simulink model "Flight_Control"  (Simulink 9.0)
settings: Solver=FixedStepDiscrete  StartTime=0.0  StopTime=tsim  FixedStep=te  RelTol=1e-3
values from neighbouring files (symbols this model uses):
  Kb_Pitch = 4    [Flight_Control_parameters.m]
  Kb_Roll = 4    [Flight_Control_parameters.m]
  Kb_Yaw = 4    [Flight_Control_parameters.m]
  Kd_Pitch = 0.037    [Flight_Control_parameters.m]
  Kd_Roll = 0.037    [Flight_Control_parameters.m]
  Kd_Yaw = 0.1    [Flight_Control_parameters.m]
  Ki_Pitch = 5    [Flight_Control_parameters.m]
  Ki_Roll = 5    [Flight_Control_parameters.m]
  Ki_Yaw = 5    [Flight_Control_parameters.m]
  Kp_Pitch = 3.84    [Flight_Control_parameters.m]
  Kp_pitch_angle = 4    [Flight_Control_parameters.m]
  Kp_Roll = 3.84    [Flight_Control_parameters.m]
  Kp_roll_angle = 4    [Flight_Control_parameters.m]
  Kp_Yaw = 8.16    [Flight_Control_parameters.m]
  te = 0.01    [Flight_Control_parameters.m]
undefined symbols (not defined in the file or in its folder): DiscIntNeverNeededParam
libraries: simulink x3
settings Model: Creator=sam  LastModifiedBy=William  ExtModeTrigDuration=2
settings DataIOCC: SaveFormat=Dataset
settings OptimizationCC: DefaultParameterBehavior=Inlined  DefaultUnderspecifiedDataType=single  PassReuseOutputArgsThreshold=0  LifeSpan=auto  MaxStackSize=64
settings DebuggingCC: UnderspecifiedInitializationDetection=Simplified  MergeDetectMultiDrivingBlocksExec=error  ParameterPrecisionLossMsg=none  ParameterTunabilityLossMsg=error
settings HardwareCC: ProdBitPerPointer=64  ProdBitPerSizeT=64  ProdBitPerPtrDiffT=64  ProdLargestAtomicFloat=Float  ProdIntDivRoundTo=Zero  ProdEndianess=LittleEndian  ProdWordSize=64  ProdHWDeviceType=Intel->x86-64 (Windows64)
settings ModelReferenceCC: PropagateSignalLabelsOutOfModel=on
settings SFSimCC: MATLABDynamicMemAlloc=off
settings RTWCC: GenerateReport=on  Toolchain=Arduino ARM  BuildConfiguration=Faster Runs  LaunchReport=on  RTWCompilerOptimization=on
settings CodeAppCC: ForceParamTrailComments=on  MaxIdLength=95  OperatorAnnotations=on  MATLABSourceComments=on
settings ConfigComp: CovScope=Subsystem  CovPath=Flight_Control  CovSaveName=covdata_decision  CovMetricSettings=dcmw  CovHTMLOptions=-sRT=1 -sVT=0 -aTS=1 -bRG=1 -bTC=1 -hTR=0 -nFC=0 -nFD=1 -scm=1 -bcm=1 -xEv=0 -xEM=0  CovNameIncrementing=on  CovOutputDir=../reports/slcov_output/$ModelName$

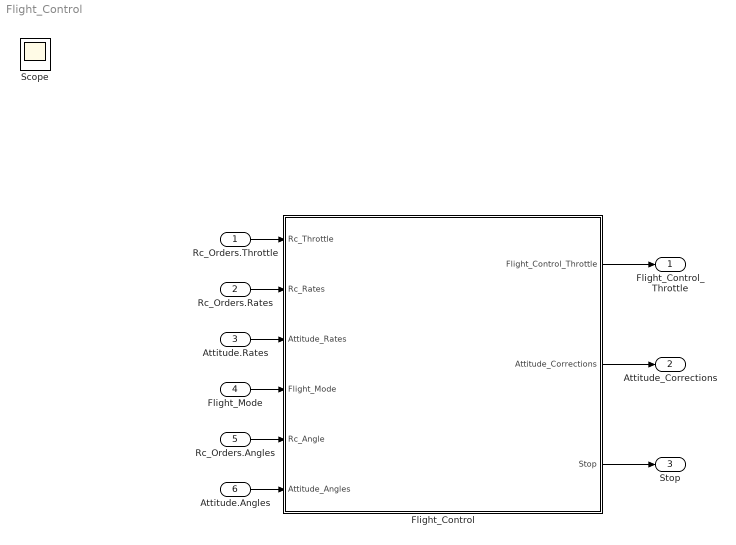
== system Flight_Control ==
  Rc_Orders.Throttle : Inport  OutDataTypeStr=single  PortDimensions=1
  Rc_Orders.Rates : Inport  Port=2  OutDataTypeStr=single  PortDimensions=3
  Attitude.Rates : Inport  Port=3  OutDataTypeStr=single  PortDimensions=3
  Flight_Mode : Inport  Port=4  OutDataTypeStr=uint8
  Rc_Orders.Angles : Inport  Port=5  OutDataTypeStr=single  PortDimensions=2
  Attitude.Angles : Inport  Port=6  OutDataTypeStr=single  PortDimensions=2
  Flight_Control : Subsystem
  Flight_Control_Throttle : Outport  OutDataTypeStr=single  PortDimensions=1
  Attitude_Corrections : Outport  Port=2  OutDataTypeStr=single  PortDimensions=3
  Stop : Outport  Port=3  OutDataTypeStr=boolean  PortDimensions=1
  Scope : Scope
  wires:
  Flight_Control/1(Flight_Control_Throttle) -> Flight_Control_Throttle/1
  Flight_Control/2(Attitude_Corrections) -> Attitude_Corrections/1
  Flight_Control/3(Stop) -> Stop/1
  Rc_Orders.Throttle/1 -> Flight_Control/1(Rc_Throttle)
  Rc_Orders.Rates/1 -> Flight_Control/2(Rc_Rates)
  Attitude.Rates/1 -> Flight_Control/3(Attitude_Rates)
  Flight_Mode/1 -> Flight_Control/4(Flight_Mode)
  Rc_Orders.Angles/1 -> Flight_Control/5(Rc_Angle)
  Attitude.Angles/1 -> Flight_Control/6(Attitude_Angles)

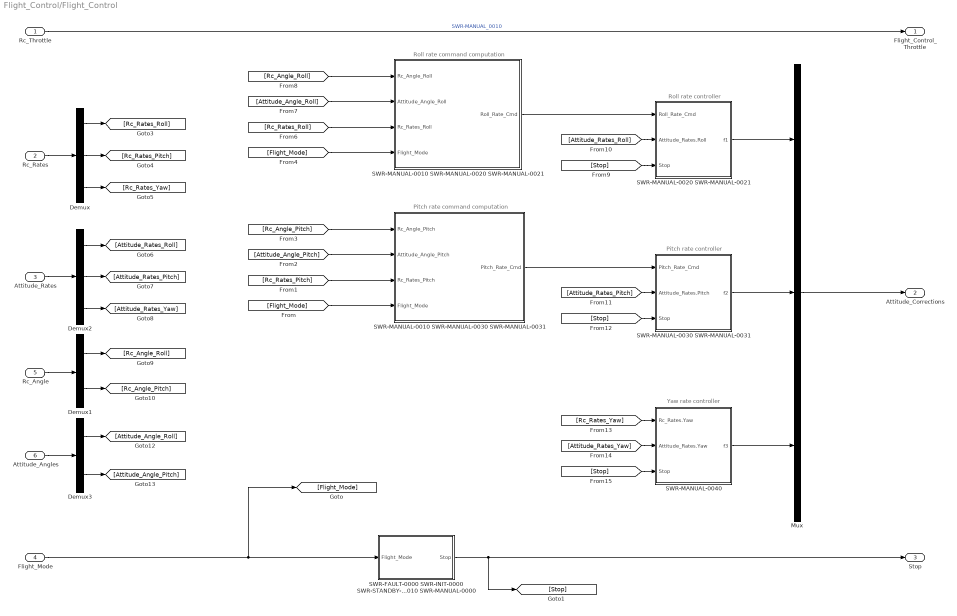
== system Flight_Control/Flight_Control ==
  note: Roll rate controller
  note: Pitch rate controller
  note: Yaw rate controller
  note: Roll rate command computation
  note: Pitch rate command computation
  Rc_Throttle : Inport  PortDimensions=1
  Rc_Rates : Inport  Port=2  PortDimensions=3
  Attitude_Rates : Inport  Port=3  PortDimensions=3
  Flight_Mode : Inport  Port=4  PortDimensions=1
  Rc_Angle : Inport  Port=5  PortDimensions=2
  Attitude_Angles : Inport  Port=6  PortDimensions=2
  Demux : Demux  Outputs=3
  Demux1 : Demux  Outputs=2
  Demux2 : Demux  Outputs=3
  Demux3 : Demux  Outputs=2
  Mux : Mux  Inputs=3
  SWR-FAULT-0000 SWR-INIT-0000 SWR-STANDBY-0000 SWR-STANDBY-0010 SWR-MANUAL-0000 : Subsystem
  "SWR-MANUAL-0010 SWR-MANUAL-0020 SWR-MANUAL-0021 " : Subsystem
  "SWR-MANUAL-0010 SWR-MANUAL-0030 SWR-MANUAL-0031 " : Subsystem
  SWR-MANUAL-0020 SWR-MANUAL-0021 : Subsystem
  SWR-MANUAL-0030 SWR-MANUAL-0031 : Subsystem
  SWR-MANUAL-0040 : Subsystem
  Flight_Control_Throttle : Outport  PortDimensions=1
  Attitude_Corrections : Outport  Port=2  PortDimensions=3
  Stop : Outport  Port=3  PortDimensions=1
  wires:
  Rc_Rates/1 -> Demux/1
  Attitude_Rates/1 -> Demux2/1
  Demux/1 -> [Rc_Rates_Roll]
  Demux/2 -> [Rc_Rates_Pitch]
  Demux/3 -> [Rc_Rates_Yaw]
  Demux2/3 -> [Attitude_Rates_Yaw]
  Demux2/1 -> [Attitude_Rates_Roll]
  Demux2/2 -> [Attitude_Rates_Pitch]
  [Attitude_Rates_Pitch] -> SWR-MANUAL-0030 SWR-MANUAL-0031/2(Attitude_Rates.Pitch)
  Mux/1 -> Attitude_Corrections/1
  SWR-FAULT-0000 SWR-INIT-0000 SWR-STANDBY-0000 SWR-STANDBY-0010 SWR-MANUAL-0000/1("Stop ") -> [Stop], Stop/1
  Rc_Throttle/1 -> Flight_Control_Throttle/1  "SWR-MANUAL_0010"
  [Stop] -> SWR-MANUAL-0020 SWR-MANUAL-0021/3(Stop)
  [Stop] -> SWR-MANUAL-0030 SWR-MANUAL-0031/3(Stop)
  SWR-MANUAL-0040/1(f3) -> Mux/3
  Rc_Angle/1 -> Demux1/1
  Demux1/1 -> [Rc_Angle_Roll]
  Demux1/2 -> [Rc_Angle_Pitch]
  Attitude_Angles/1 -> Demux3/1
  Demux3/2 -> [Attitude_Angle_Pitch]
  Demux3/1 -> [Attitude_Angle_Roll]
  [Attitude_Rates_Roll] -> SWR-MANUAL-0020 SWR-MANUAL-0021/2(Attitude_Rates.Roll)
  Flight_Mode/1 -> SWR-FAULT-0000 SWR-INIT-0000 SWR-STANDBY-0000 SWR-STANDBY-0010 SWR-MANUAL-0000/1(Flight_Mode), [Flight_Mode]
  SWR-MANUAL-0020 SWR-MANUAL-0021/1(f1) -> Mux/1
  SWR-MANUAL-0030 SWR-MANUAL-0031/1(f2) -> Mux/2
  [Rc_Rates_Yaw] -> SWR-MANUAL-0040/1(Rc_Rates.Yaw)
  [Attitude_Rates_Yaw] -> SWR-MANUAL-0040/2(Attitude_Rates.Yaw)
  [Stop] -> SWR-MANUAL-0040/3(Stop)
  "SWR-MANUAL-0010 SWR-MANUAL-0020 SWR-MANUAL-0021 "/1(Roll_Rate_Cmd) -> SWR-MANUAL-0020 SWR-MANUAL-0021/1(Roll_Rate_Cmd)
  [Rc_Angle_Roll] -> "SWR-MANUAL-0010 SWR-MANUAL-0020 SWR-MANUAL-0021 "/1(Rc_Angle_Roll)
  [Attitude_Angle_Roll] -> "SWR-MANUAL-0010 SWR-MANUAL-0020 SWR-MANUAL-0021 "/2(Attitude_Angle_Roll)
  [Flight_Mode] -> "SWR-MANUAL-0010 SWR-MANUAL-0020 SWR-MANUAL-0021 "/4(Flight_Mode)
  [Rc_Rates_Roll] -> "SWR-MANUAL-0010 SWR-MANUAL-0020 SWR-MANUAL-0021 "/3(Rc_Rates_Roll)
  "SWR-MANUAL-0010 SWR-MANUAL-0030 SWR-MANUAL-0031 "/1(Pitch_Rate_Cmd) -> SWR-MANUAL-0030 SWR-MANUAL-0031/1(Pitch_Rate_Cmd)
  [Rc_Angle_Pitch] -> "SWR-MANUAL-0010 SWR-MANUAL-0030 SWR-MANUAL-0031 "/1(Rc_Angle_Pitch)
  [Attitude_Angle_Pitch] -> "SWR-MANUAL-0010 SWR-MANUAL-0030 SWR-MANUAL-0031 "/2(Attitude_Angle_Pitch)
  [Rc_Rates_Pitch] -> "SWR-MANUAL-0010 SWR-MANUAL-0030 SWR-MANUAL-0031 "/3(Rc_Rates_Pitch)
  [Flight_Mode] -> "SWR-MANUAL-0010 SWR-MANUAL-0030 SWR-MANUAL-0031 "/4(Flight_Mode)

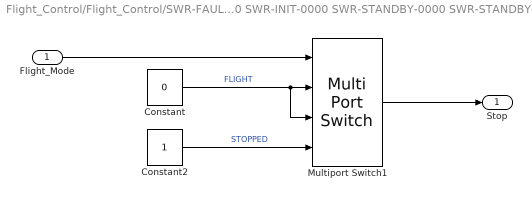
== system Flight_Control/Flight_Control/SWR-FAULT-0000 SWR-INIT-0000 SWR-STANDBY-0000 SWR-STANDBY-0010 SWR-MANUAL-0000 ==
  Flight_Mode : Inport  PortDimensions=1
  Constant : Constant  Value=0  OutDataTypeStr=boolean
  Constant2 : Constant  OutDataTypeStr=boolean
  Multiport Switch1 : MultiPortSwitch  DiagnosticForDefault=None
  "Stop " : Outport  PortDimensions=1
  wires:
  Constant/1 -> Multiport Switch1/3, Multiport Switch1/2  "FLIGHT"
  Flight_Mode/1 -> Multiport Switch1/1
  Multiport Switch1/1 -> "Stop "/1
  Constant2/1 -> Multiport Switch1/4  "STOPPED"

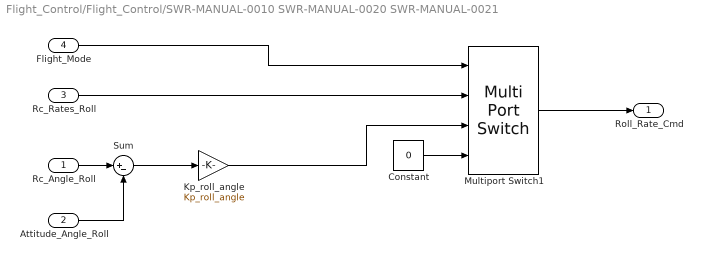
== system Flight_Control/Flight_Control/SWR-MANUAL-0010 SWR-MANUAL-0020 SWR-MANUAL-0021  ==
  Rc_Angle_Roll : Inport
  Attitude_Angle_Roll : Inport  Port=2
  Rc_Rates_Roll : Inport  Port=3
  Flight_Mode : Inport  Port=4
  Constant : Constant  Value=0  OutDataTypeStr=single
  Kp_roll_angle : Gain  Gain=Kp_roll_angle
  Multiport Switch1 : MultiPortSwitch  DiagnosticForDefault=None
  Sum : Sum  Inputs=|+-
  Roll_Rate_Cmd : Outport
  wires:
  Multiport Switch1/1 -> Roll_Rate_Cmd/1
  Kp_roll_angle/1 -> Multiport Switch1/3
  Rc_Angle_Roll/1 -> Sum/1
  Attitude_Angle_Roll/1 -> Sum/2
  Sum/1 -> Kp_roll_angle/1
  Flight_Mode/1 -> Multiport Switch1/1
  Rc_Rates_Roll/1 -> Multiport Switch1/2
  Constant/1 -> Multiport Switch1/4

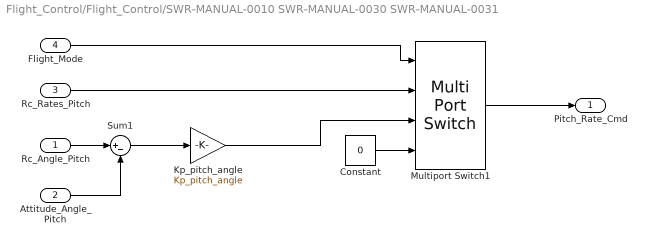
== system Flight_Control/Flight_Control/SWR-MANUAL-0010 SWR-MANUAL-0030 SWR-MANUAL-0031  ==
  Rc_Angle_Pitch : Inport
  Attitude_Angle_Pitch : Inport  Port=2
  Rc_Rates_Pitch : Inport  Port=3
  Flight_Mode : Inport  Port=4
  Constant : Constant  Value=0  OutDataTypeStr=single
  Kp_pitch_angle : Gain  Gain=Kp_pitch_angle
  Multiport Switch1 : MultiPortSwitch  DiagnosticForDefault=None
  Sum1 : Sum  Inputs=|+-
  Pitch_Rate_Cmd : Outport
  wires:
  Sum1/1 -> Kp_pitch_angle/1
  Rc_Angle_Pitch/1 -> Sum1/1
  Attitude_Angle_Pitch/1 -> Sum1/2
  Multiport Switch1/1 -> Pitch_Rate_Cmd/1
  Flight_Mode/1 -> Multiport Switch1/1
  Rc_Rates_Pitch/1 -> Multiport Switch1/2
  Kp_pitch_angle/1 -> Multiport Switch1/3
  Constant/1 -> Multiport Switch1/4

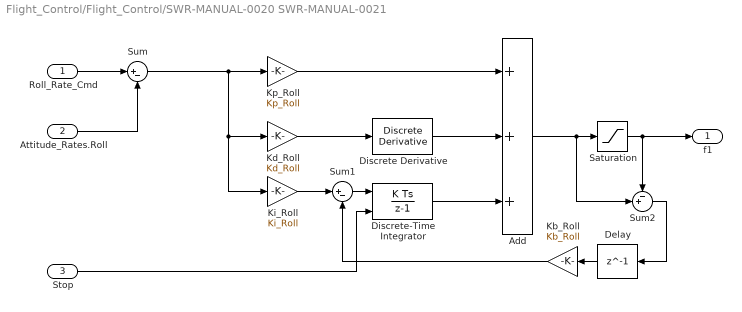
== system Flight_Control/Flight_Control/SWR-MANUAL-0020 SWR-MANUAL-0021 ==
  Roll_Rate_Cmd : Inport  PortDimensions=1
  Attitude_Rates.Roll : Inport  Port=2  PortDimensions=1
  Stop : Inport  Port=3  PortDimensions=1
  Add : Sum  Inputs=+++
  Delay : Delay  DelayLength=1  InitialCondition=0  SampleTime=te
  Discrete Derivative : simulink/Discrete/Discrete Derivative  gainval=1.0  ICPrevScaledInput=0.0  OutMin=[]  OutMax=[]  OutDataType=fixdt(1, 16)  OutScaling=2^-10  DoSatur=off
  Discrete-Time Integrator : DiscreteIntegrator  ExternalReset=level  InitialConditionSetting=State (most efficient)  SampleTime=te  UpperSaturationLimit=100  LowerSaturationLimit=-100  ICPrevOutput=DiscIntNeverNeededParam  ICPrevScaledInput=DiscIntNeverNeededParam
  Kb_Roll : Gain  Gain=Kb_Roll  ParamDataTypeStr=Inherit: Same as input
  Kd_Roll : Gain  Gain=Kd_Roll  ParamDataTypeStr=Inherit: Same as input
  Ki_Roll : Gain  Gain=Ki_Roll  ParamDataTypeStr=Inherit: Same as input
  Kp_Roll : Gain  Gain=Kp_Roll  ParamDataTypeStr=Inherit: Same as input
  Saturation : Saturate  UpperLimit=30  LowerLimit=-30
  Sum : Sum  Inputs=|+-
  Sum1 : Sum  Inputs=|+-
  Sum2 : Sum  Inputs=-+|
  f1 : Outport  PortDimensions=1
  wires:
  Add/1 -> Saturation/1, Sum2/2
  Roll_Rate_Cmd/1 -> Sum/1
  Attitude_Rates.Roll/1 -> Sum/2
  Sum/1 -> Kd_Roll/1, Ki_Roll/1, Kp_Roll/1
  Kp_Roll/1 -> Add/1
  Stop/1 -> Discrete-Time Integrator/2
  Discrete-Time Integrator/1 -> Add/3
  Discrete Derivative/1 -> Add/2
  Kd_Roll/1 -> Discrete Derivative/1
  Saturation/1 -> f1/1, Sum2/1
  Sum2/1 -> Delay/1
  Delay/1 -> Kb_Roll/1
  Kb_Roll/1 -> Sum1/2
  Sum1/1 -> Discrete-Time Integrator/1
  Ki_Roll/1 -> Sum1/1

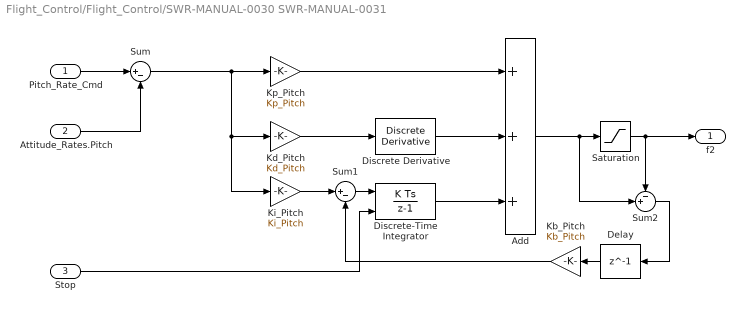
== system Flight_Control/Flight_Control/SWR-MANUAL-0030 SWR-MANUAL-0031 ==
  Pitch_Rate_Cmd : Inport  PortDimensions=1
  Attitude_Rates.Pitch : Inport  Port=2  PortDimensions=1
  Stop : Inport  Port=3  PortDimensions=1
  Add : Sum  Inputs=+++
  Delay : Delay  DelayLength=1  InitialCondition=0  SampleTime=te
  Discrete Derivative : simulink/Discrete/Discrete Derivative  gainval=1.0  ICPrevScaledInput=0.0  OutMin=[]  OutMax=[]  OutDataType=fixdt(1, 16)  OutScaling=2^-10  DoSatur=off
  Discrete-Time Integrator : DiscreteIntegrator  ExternalReset=level  InitialConditionSetting=State (most efficient)  SampleTime=te  UpperSaturationLimit=100  LowerSaturationLimit=-100  ICPrevOutput=DiscIntNeverNeededParam  ICPrevScaledInput=DiscIntNeverNeededParam
  Kb_Pitch : Gain  Gain=Kb_Pitch  ParamDataTypeStr=Inherit: Same as input
  Kd_Pitch : Gain  Gain=Kd_Pitch  ParamDataTypeStr=Inherit: Same as input
  Ki_Pitch : Gain  Gain=Ki_Pitch  ParamDataTypeStr=Inherit: Same as input
  Kp_Pitch : Gain  Gain=Kp_Pitch  ParamDataTypeStr=Inherit: Same as input
  Saturation : Saturate  UpperLimit=30  LowerLimit=-30
  Sum : Sum  Inputs=|+-
  Sum1 : Sum  Inputs=|+-
  Sum2 : Sum  Inputs=-+|
  f2 : Outport  PortDimensions=1
  wires:
  Add/1 -> Saturation/1, Sum2/2
  Pitch_Rate_Cmd/1 -> Sum/1
  Attitude_Rates.Pitch/1 -> Sum/2
  Sum/1 -> Kd_Pitch/1, Ki_Pitch/1, Kp_Pitch/1
  Kp_Pitch/1 -> Add/1
  Stop/1 -> Discrete-Time Integrator/2
  Discrete-Time Integrator/1 -> Add/3
  Discrete Derivative/1 -> Add/2
  Kd_Pitch/1 -> Discrete Derivative/1
  Saturation/1 -> f2/1, Sum2/1
  Sum2/1 -> Delay/1
  Delay/1 -> Kb_Pitch/1
  Kb_Pitch/1 -> Sum1/2
  Sum1/1 -> Discrete-Time Integrator/1
  Ki_Pitch/1 -> Sum1/1

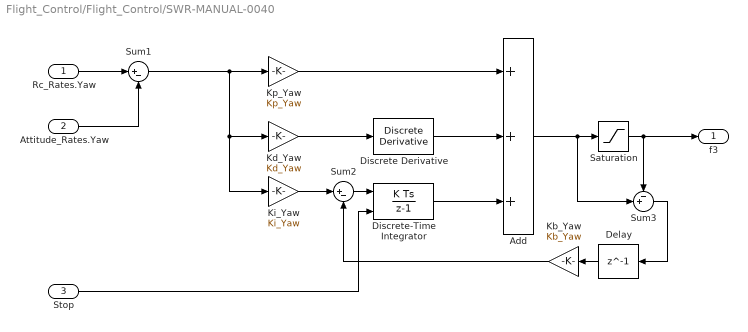
== system Flight_Control/Flight_Control/SWR-MANUAL-0040 ==
  Rc_Rates.Yaw : Inport  PortDimensions=1
  Attitude_Rates.Yaw : Inport  Port=2  PortDimensions=1
  Stop : Inport  Port=3  PortDimensions=1
  Add : Sum  Inputs=+++
  Delay : Delay  DelayLength=1  InitialCondition=0  SampleTime=te
  Discrete Derivative : simulink/Discrete/Discrete Derivative  gainval=1.0  ICPrevScaledInput=0.0  OutMin=[]  OutMax=[]  OutDataType=fixdt(1, 16)  OutScaling=2^-10  DoSatur=off
  Discrete-Time Integrator : DiscreteIntegrator  ExternalReset=level  InitialConditionSetting=State (most efficient)  SampleTime=te  UpperSaturationLimit=100  LowerSaturationLimit=-100  ICPrevOutput=DiscIntNeverNeededParam  ICPrevScaledInput=DiscIntNeverNeededParam
  Kb_Yaw : Gain  Gain=Kb_Yaw  ParamDataTypeStr=Inherit: Same as input
  Kd_Yaw : Gain  Gain=Kd_Yaw  ParamDataTypeStr=Inherit: Same as input
  Ki_Yaw : Gain  Gain=Ki_Yaw  ParamDataTypeStr=Inherit: Same as input
  Kp_Yaw : Gain  Gain=Kp_Yaw  ParamDataTypeStr=Inherit: Same as input
  Saturation : Saturate  UpperLimit=30  LowerLimit=-30
  Sum1 : Sum  Inputs=|+-
  Sum2 : Sum  Inputs=|+-
  Sum3 : Sum  Inputs=-+|
  f3 : Outport  PortDimensions=1
  wires:
  Discrete-Time Integrator/1 -> Add/3
  Sum1/1 -> Kd_Yaw/1, Ki_Yaw/1, Kp_Yaw/1
  Ki_Yaw/1 -> Sum2/1
  Saturation/1 -> f3/1, Sum3/1
  Kb_Yaw/1 -> Sum2/2
  Delay/1 -> Kb_Yaw/1
  Rc_Rates.Yaw/1 -> Sum1/1
  Kp_Yaw/1 -> Add/1
  Kd_Yaw/1 -> Discrete Derivative/1
  Sum3/1 -> Delay/1
  Add/1 -> Saturation/1, Sum3/2
  Discrete Derivative/1 -> Add/2
  Sum2/1 -> Discrete-Time Integrator/1
  Stop/1 -> Discrete-Time Integrator/2
  Attitude_Rates.Yaw/1 -> Sum1/2
